simulink model "delaybug"  (Simulink 6.2)
settings: Solver=ode4  SolverMode=SingleTasking  StartTime=0.0  StopTime=1.5  FixedStep=.001  RelTol=1e-3  AbsTol=1e-6
settings Model: Creator=jacobs  LastModifiedBy=jacobs  ExtModeAutoUpdateStatusClock=off
settings DataIOCC: LimitDataPoints=off
settings OptimizationCC: BlockReduction=off  BooleanDataType=off
settings HardwareCC: TargetUnknown=on
settings GRTTargetCC: ModelReferenceCompliant=off  MatFileLogging=off

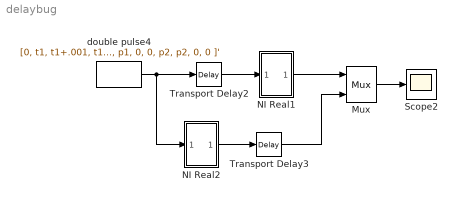
== system delaybug ==
  Mux : Mux  Inputs=2
  NI Real1 : Subsystem
      mask Display: disp('NI\nReal')
  NI Real2 : Subsystem
      mask Display: disp('NI\nReal')
  Scope2 : Scope
      settings: TickLabels=on  TimeRange=1.5  YMin=0  YMax=1  DataFormat=Array
  Transport Delay2 : TransportDelay  DelayTime=0.022
      mask Display: disp('22ms')
  Transport Delay3 : TransportDelay  DelayTime=0.022
      mask Display: disp('22ms')
  double pulse4 : FromWorkspace  VariableName=[0, t1, t1+.001, t1+d1, t1+d1+.001, t1+d1+.001+ipd, t1+d1+.001+ipd, t1+d1+.001+ipd+d2, t1+d1+.001+ipd+d2, 10000; 0, 0, p1, p1, 0, 0, p2, p2, 0, 0 ]'  SampleTime=.001  mask{@1=15, @2=.25, @3=.25, @4=0, @5=0, @6=0}
      mask prompts: @1 "Pulse 1 Magnitude"; @2 "Time of Pulse 1 Onset"; @3 "Pulse 1 Duration"; @4 "Interpulse Delay"; @5 "Pulse 2 Magnitude"; @6 "Pulse 2 Duration"
      mask help: Double Pulse
      mask init:
      | p1=@1; t1=@2; d1=@3; ipd=@4; p2=@5; d2=@6;
      mask Display: disp('Double\nPulse')
  wires:
  Transport Delay2/1 -> NI Real1/1(PG + (TIAL+SP))
  NI Real2/1(NIOUT [epospr]) -> Transport Delay3/1
  NI Real1/1(NIOUT [epospr]) -> Mux/1
  double pulse4/1 -> Transport Delay2/1, NI Real2/1(PG + (TIAL+SP))
  Transport Delay3/1 -> Mux/2
  Mux/1 -> Scope2/1

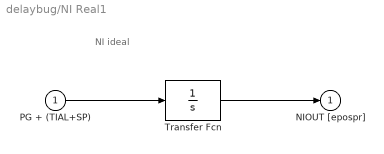
== system delaybug/NI Real1 ==
  note: NI ideal
  PG + (TIAL+SP) : Inport  Port=1  LatchInput=off
  Transfer Fcn : TransferFcn  Numerator=1  Denominator=[1 0]
  NIOUT [epospr] : Outport  InitialOutput=0
  wires:
  Transfer Fcn/1 -> NIOUT [epospr]/1
  PG + (TIAL+SP)/1 -> Transfer Fcn/1

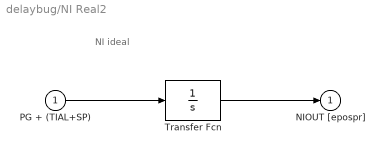
== system delaybug/NI Real2 ==
  note: NI ideal
  PG + (TIAL+SP) : Inport  Port=1  LatchInput=off
  Transfer Fcn : TransferFcn  Numerator=1  Denominator=[1 0]
  NIOUT [epospr] : Outport  InitialOutput=0
  wires:
  Transfer Fcn/1 -> NIOUT [epospr]/1
  PG + (TIAL+SP)/1 -> Transfer Fcn/1
